simulink model "Cycle_closed_loop"  (R2020b)
settings: Solver=FixedStepAuto  StartTime=0.0  StopTime=inf  RelTol=1e-3  EnableMultiTasking=on
libraries: arduinomotorcarrierlib x2, eeGeneralControl x1, arduinosensorlib x1
settings Model: SimulationMode=external  SILPILModeSetting=veronly  ExtModeTrigDuration=2  Creator=bkhusain  LastModifiedBy=gbellido
settings OptimizationCC: EnhancedBackFolding=on  PassReuseOutputArgsAs=Individual arguments  ZeroExternalMemoryAtStartup=off  ZeroInternalMemoryAtStartup=off  MaxStackSize=64  OptimizeBlockOrder=speed  DifferentSizesBufferReuse=on  OptimizationCustomize=off  EfficientTunableParamExpr=on
settings DebuggingCC: ParameterTunabilityLossMsg=error
settings HardwareCC: ProdBitPerPointer=32  ProdBitPerSizeT=32  ProdBitPerPtrDiffT=32  ProdLargestAtomicInteger=Long  ProdLargestAtomicFloat=Double  ProdWordSize=32  ProdHWDeviceType=ARM Compatible->ARM Cortex  UseEmbeddedCoderFeatures=off  UseSimulinkCoderFeatures=off
settings SFSimCC: MATLABDynamicMemAlloc=off
settings RTWCC: Description=Embedded Coder  SystemTargetFile=ert.tlc  HardwareBoard=Arduino Nano 33 IoT  TemplateMakefile=ert_default_tmf  Toolchain=Arduino ARM  BuildConfiguration=Faster Runs
settings CodeAppCC: ForceParamTrailComments=on  IgnoreCustomStorageClasses=off  OperatorAnnotations=on  SimulinkDataObjDesc=on  SFDataObjDesc=on  MangleLength=10  InsertBlockDesc=on
settings ERTTargetCC: SupportContinuousTime=on  SupportNonInlinedSFcns=on  SupportVariableSizeSignals=on  ExtModeStaticAllocSize=8192

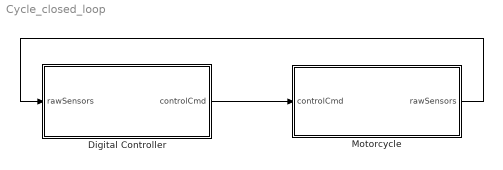
== system Cycle_closed_loop ==
  Digital Controller : Subsystem
  Motorcycle : Subsystem
  wires:
  Digital Controller/1(controlCmd) -> Motorcycle/1(controlCmd)
  Motorcycle/1(rawSensors) -> Digital Controller/1(rawSensors)

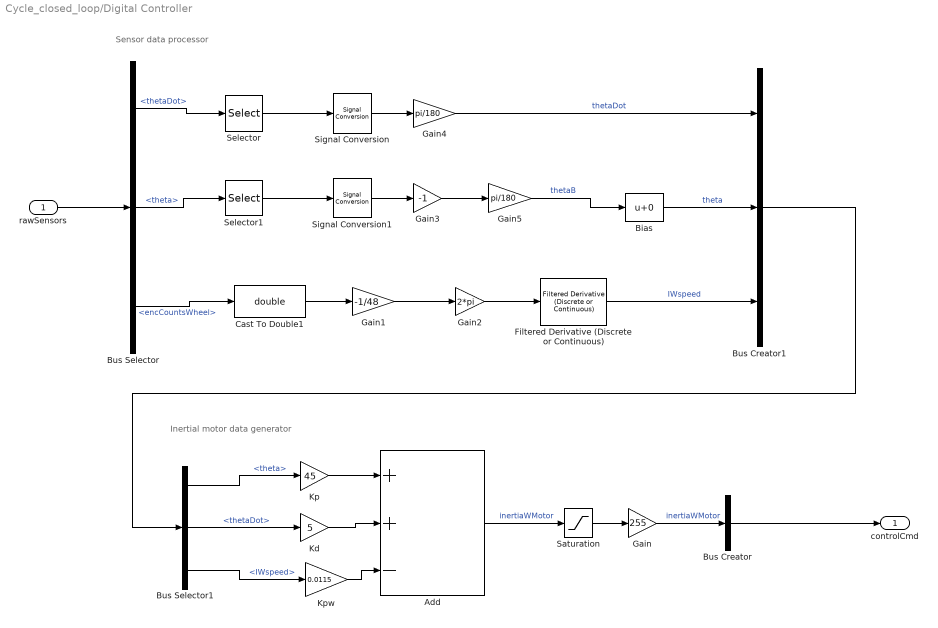
== system Cycle_closed_loop/Digital Controller ==
  note: Inertial motor data generator
  note: Sensor data processor
  rawSensors : Inport
  Add : Sum  Inputs=++-
  Bias : Bias
  Bus Creator : BusCreator  Inputs=1
  Bus Creator1 : BusCreator  Inputs=3
  Bus Selector : BusSelector  OutputSignals=thetaDot,theta,encCountsWheel
  Bus Selector1 : BusSelector  OutputSignals=theta,thetaDot,IWspeed
  Cast To Double1 : DataTypeConversion  OutDataTypeStr=double
  Filtered Derivative (Discrete or Continuous) : eeGeneralControl/Filtered Derivative (Discrete or Continuous)  K=1  T=0.1  B=inf  A=-inf  minRatio=10  init_option=Inherited from block input  x0=0  Ts=0.01
      settings: SourceProductBaseCode=PS
  Gain : Gain  Gain=255
  Gain1 : Gain  Gain=-1/48
  Gain2 : Gain  Gain=2*pi
  Gain3 : Gain  Gain=-1
  Gain4 : Gain  Gain=pi/180
  Gain5 : Gain  Gain=pi/180
  Kd : Gain  Gain=5
  Kp : Gain  Gain=45
  Kpw : Gain  Gain=0.0115
  Saturation : Saturate  UpperLimit=1  LowerLimit=-1
  Selector : Selector  InputPortWidth=3  IndexOptions=Index vector (dialog)  Indices=[2]  OutputSizes=1
  Selector1 : Selector  InputPortWidth=3  IndexOptions=Index vector (dialog)  Indices=[2]  OutputSizes=1
  Signal Conversion : SignalConversion  OverrideOpt=off
  Signal Conversion1 : SignalConversion  OverrideOpt=off
  controlCmd : Outport
  wires:
  Bus Creator/1 -> controlCmd/1
  Add/1 -> Saturation/1  "inertiaWMotor"
  Saturation/1 -> Gain/1
  Gain/1 -> Bus Creator/1  "inertiaWMotor"
  Bias/1 -> Bus Creator1/2  "theta"
  Gain4/1 -> Bus Creator1/1  "thetaDot"
  Signal Conversion/1 -> Gain4/1
  Gain2/1 -> Filtered Derivative (Discrete or Continuous)/1
  Bus Selector/3 -> Cast To Double1/1  "<encCountsWheel>"
  Bus Selector/2 -> Selector1/1  "<theta>"
  Gain3/1 -> Gain5/1
  Filtered Derivative (Discrete or Continuous)/1 -> Bus Creator1/3  "IWspeed"
  Gain5/1 -> Bias/1  "thetaB"
  Selector/1 -> Signal Conversion/1
  Cast To Double1/1 -> Gain1/1
  rawSensors/1 -> Bus Selector/1
  Gain1/1 -> Gain2/1
  Selector1/1 -> Signal Conversion1/1
  Bus Selector/1 -> Selector/1  "<thetaDot>"
  Signal Conversion1/1 -> Gain3/1
  Bus Selector1/3 -> Kpw/1  "<IWspeed>"
  Bus Selector1/2 -> Kd/1  "<thetaDot>"
  Bus Selector1/1 -> Kp/1  "<theta>"
  Kp/1 -> Add/1
  Kd/1 -> Add/2
  Kpw/1 -> Add/3
  Bus Creator1/1 -> Bus Selector1/1

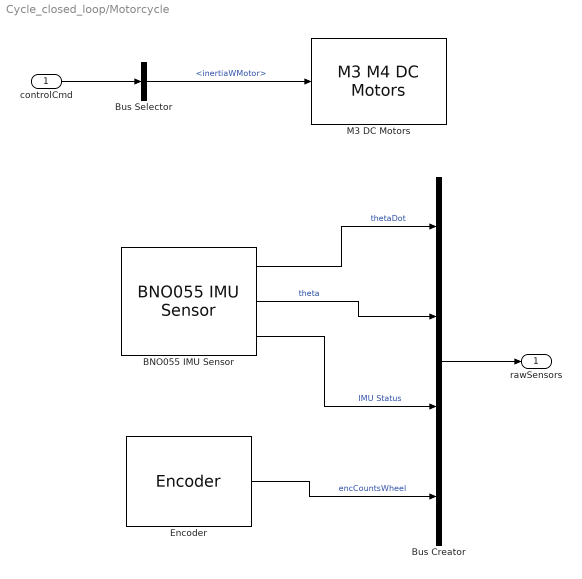
== system Cycle_closed_loop/Motorcycle ==
  controlCmd : Inport
  BNO055 IMU Sensor : arduinosensorlib/BNO055 IMU Sensor  SlaveAddress=0x28  OperationMode=Fusion  Accel=off  AngularRate=on  MagField=off  EulerAngles=on  Quat=off  LinearAccel=off  GravityVector=off  AccelRange=4G  AccelBW=62.5 Hz  GyroRange=2000 dps  GyroBW=32 Hz  MagODR=10 Hz  SampleTime=0.01  blockPlatform=ARDUINO
      settings: SourceProductBaseCode=ARDUINO
  Bus Creator : BusCreator  Inputs=4
  Bus Selector : BusSelector  OutputSignals=inertiaWMotor
  Encoder : arduinomotorcarrierlib/Encoder  SlaveAddress=uint8( hex2dec( '66' ) )  blockPlatform=ARDUINO  Encoder=1  ShowSpeed=off  ResetOption=on  SampleTime=0.01
      settings: SourceProductBaseCode=ARDUINO
  M3 DC Motors : arduinomotorcarrierlib/M3 M4 DC Motors  MotorNumber=M3  forwardPinNumber=3  reversePinNumber=2
      settings: SourceProductBaseCode=ARDUINO
  rawSensors : Outport
  wires:
  BNO055 IMU Sensor/1 -> Bus Creator/1  "thetaDot"
  BNO055 IMU Sensor/2 -> Bus Creator/2  "theta"
  BNO055 IMU Sensor/3 -> Bus Creator/3  "IMU Status"
  Encoder/1 -> Bus Creator/4  "encCountsWheel"
  Bus Creator/1 -> rawSensors/1
  controlCmd/1 -> Bus Selector/1
  Bus Selector/1 -> M3 DC Motors/1  "<inertiaWMotor>"
